simulink model "elsayed"  (R2023a)
settings: Solver=ode45  StartTime=0.0  StopTime=360  MaxStep=7.2  RelTol=1e-3
settings Model: Creator=Dell  LastModifiedBy=ENG-ELSAYED
settings SolverCC: MaxConsecutiveMinStep=10  AlgebraicLoopSolver=TrustRegion
settings DataIOCC: ReturnWorkspaceOutputs=off
settings DebuggingCC: UnconnectedInputMsg=warning  UnconnectedOutputMsg=warning  UnconnectedLineMsg=warning  ArithmeticOperatorsInVariantConditions=warning
settings ModelReferenceCC: EnableRefExpFcnMdlSchedulingChecks=on
settings SFSimCC: SimUseLocalCustomCode=off  CustomCodeUndefinedFunction=UseInterfaceOnly
settings RTWCC: RTWUseLocalCustomCode=off  DLArmComputeVersion=19.05

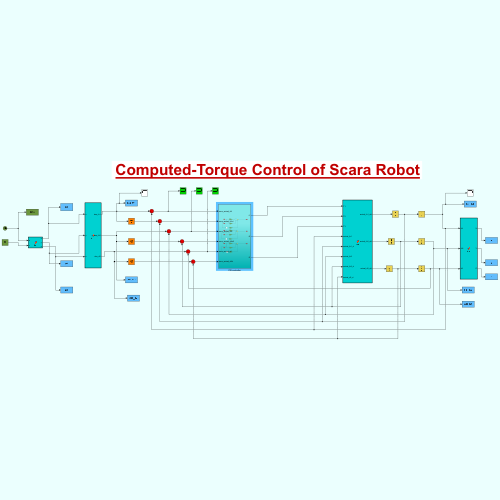
[thumbnail: Simulink's stored preview of the top-level diagram]
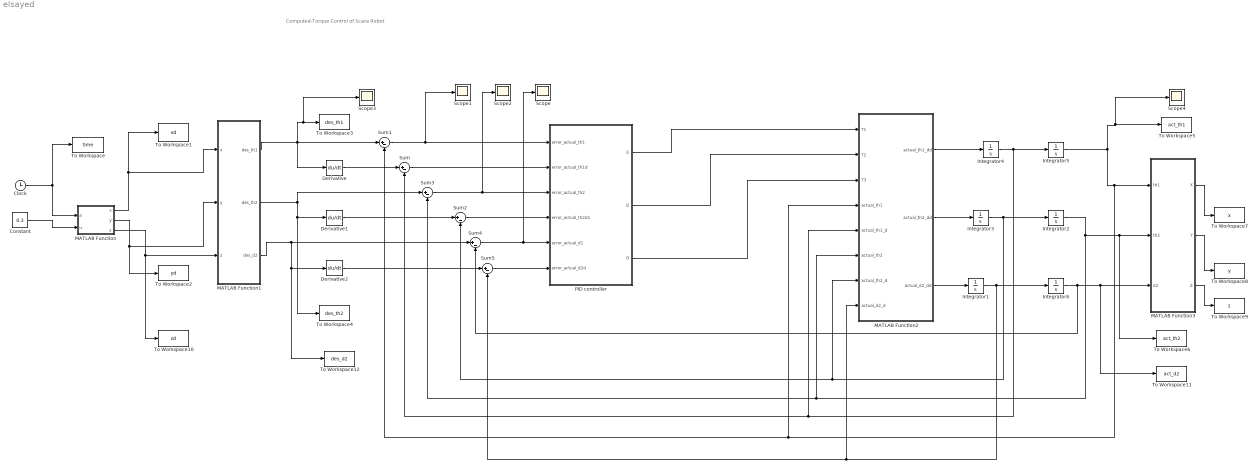
== system elsayed ==
  note: Computed-Torque Control of Scara Robot
  Clock : Clock
  Constant : Constant  Value=0.3
  Derivative : Derivative
  Derivative1 : Derivative
  Derivative2 : Derivative
  Integrator{1..6} (6 alike) : Integrator
  MATLAB Function : MATLAB Function  TreatAsAtomicUnit=on
  MATLAB Function1 : MATLAB Function  TreatAsAtomicUnit=on
  MATLAB Function2 : MATLAB Function  TreatAsAtomicUnit=on
  MATLAB Function3 : MATLAB Function  TreatAsAtomicUnit=on
  PID controller : Subsystem
  Scope{,1..4} (5 alike) : Scope
  Sum{,1..5} (6 alike) : Sum  Inputs=|+-
  To Workspace : ToWorkspace  VariableName=time  SampleTime=-1
  To Workspace1 : ToWorkspace  VariableName=xd  SampleTime=-1
  To Workspace10 : ToWorkspace  VariableName=zd  SampleTime=-1
      settings: Save2DSignal=2-D array (concatenate along first dimension)
  To Workspace11 : ToWorkspace  VariableName=act_d2  SampleTime=-1
  To Workspace12 : ToWorkspace  VariableName=des_d2  SampleTime=-1
  To Workspace2 : ToWorkspace  VariableName=yd  SampleTime=-1
      settings: Save2DSignal=2-D array (concatenate along first dimension)
  To Workspace3 : ToWorkspace  VariableName=des_th1  SampleTime=-1
  To Workspace4 : ToWorkspace  VariableName=des_th2  SampleTime=-1
  To Workspace5 : ToWorkspace  VariableName=act_th1  SampleTime=-1
  To Workspace6 : ToWorkspace  VariableName=act_th2  SampleTime=-1
  To Workspace7 : ToWorkspace  VariableName=x  SampleTime=-1
  To Workspace8 : ToWorkspace  VariableName=y  SampleTime=-1
  To Workspace9 : ToWorkspace  VariableName=z  SampleTime=-1
  wires:
  Clock/1 -> MATLAB Function/1(a), To Workspace/1
  MATLAB Function/1(x) -> MATLAB Function1/1(x), To Workspace1/1
  MATLAB Function/2(y) -> MATLAB Function1/2(y), To Workspace2/1
  MATLAB Function1/2(des_th2) -> To Workspace4/1, Derivative1/1, Sum3/1
  Derivative/1 -> Sum/1
  Derivative1/1 -> Sum2/1
  Sum/1 -> PID controller/2(error_actual_th1d)
  Sum3/1 -> Scope2/1, PID controller/3(error_actual_th2)
  Sum2/1 -> PID controller/4(error_actual_th2d1)
  PID controller/1(i1) -> MATLAB Function2/1(T1)
  PID controller/2(i2) -> MATLAB Function2/2(T2)
  MATLAB Function2/2(actual_th2_dd) -> Integrator3/1
  Integrator4/1 -> MATLAB Function2/5(actual_th1_d), Sum/2, Integrator5/1
  Integrator3/1 -> MATLAB Function2/7(actual_th2_d), Sum2/2, Integrator2/1
  Integrator5/1 -> MATLAB Function2/4(actual_th1), Sum1/2, MATLAB Function3/1(th1), Scope4/1, To Workspace5/1
  Integrator2/1 -> MATLAB Function2/6(actual_th2), Sum3/2, To Workspace6/1, MATLAB Function3/2(th2)
  MATLAB Function3/1(X) -> To Workspace7/1
  Sum1/1 -> Scope1/1, PID controller/1(error_actual_th1)
  Constant/1 -> MATLAB Function/2(u)
  MATLAB Function2/1(actual_th1_dd) -> Integrator4/1
  Sum4/1 -> Scope/1, PID controller/5(error_actual_d1)
  Derivative2/1 -> Sum5/1
  Sum5/1 -> PID controller/6(error_actual_d2d)
  PID controller/3(i3) -> MATLAB Function2/3(T3)
  MATLAB Function2/3(actual_d2_dd) -> Integrator1/1
  Integrator6/1 -> Sum4/2, To Workspace11/1, MATLAB Function3/3(d2)
  Integrator1/1 -> MATLAB Function2/8(actual_d2_d), Sum5/2, Integrator6/1
  MATLAB Function3/3(Z) -> To Workspace9/1
  MATLAB Function/3(z) -> MATLAB Function1/3(z), To Workspace10/1
  MATLAB Function1/1(des_th1) -> Derivative/1, Sum1/1, Scope3/1, To Workspace3/1
  MATLAB Function3/2(Y) -> To Workspace8/1
  MATLAB Function1/3(des_d2) -> To Workspace12/1, Derivative2/1, Sum4/1

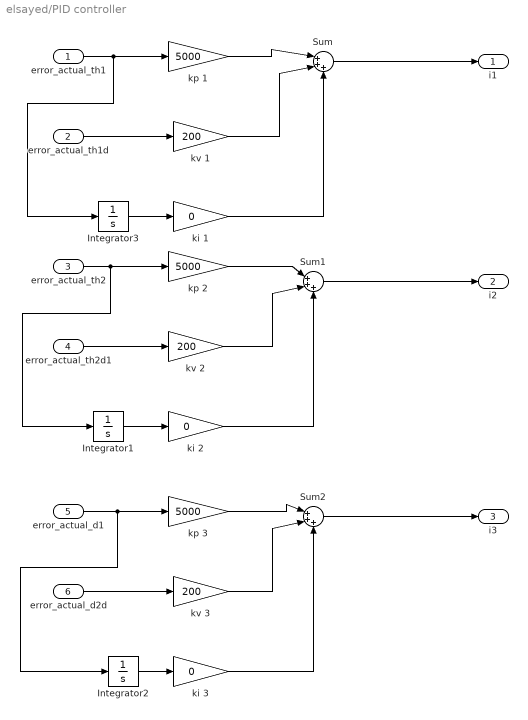
== system elsayed/PID controller ==
  error_actual_th1 : Inport
  error_actual_th1d : Inport  Port=2
  error_actual_th2 : Inport  Port=3
  error_actual_th2d1 : Inport  Port=4
  error_actual_d1 : Inport  Port=5
  error_actual_d2d : Inport  Port=6
  Integrator1 : Integrator
  Integrator2 : Integrator
  Integrator3 : Integrator
  Sum : Sum  Inputs=|+++
  Sum1 : Sum  Inputs=|+++
  Sum2 : Sum  Inputs=|+++
  ki 1 : Gain  Gain=0
  ki 2 : Gain  Gain=0
  ki 3 : Gain  Gain=0
  kp 1 : Gain  Gain=5000
  kp 2 : Gain  Gain=5000
  kp 3 : Gain  Gain=5000
  kv 1 : Gain  Gain=200
  kv 2 : Gain  Gain=200
  kv 3 : Gain  Gain=200
  i1 : Outport  VectorParamsAs1DForOutWhenUnconnected=off
  i2 : Outport  Port=2  VectorParamsAs1DForOutWhenUnconnected=off
  i3 : Outport  Port=3  VectorParamsAs1DForOutWhenUnconnected=off
  wires:
  Sum1/1 -> i2/1
  kp 2/1 -> Sum1/1
  kv 2/1 -> Sum1/2
  Sum2/1 -> i3/1
  kv 3/1 -> Sum2/2
  kp 3/1 -> Sum2/1
  Sum/1 -> i1/1
  kv 1/1 -> Sum/2
  kp 1/1 -> Sum/1
  error_actual_th1d/1 -> kv 1/1
  error_actual_th2d1/1 -> kv 2/1
  error_actual_d2d/1 -> kv 3/1
  Integrator1/1 -> ki 2/1
  error_actual_th2/1 -> Integrator1/1, kp 2/1
  ki 2/1 -> Sum1/3
  error_actual_d1/1 -> Integrator2/1, kp 3/1
  Integrator2/1 -> ki 3/1
  ki 3/1 -> Sum2/3
  Integrator3/1 -> ki 1/1
  error_actual_th1/1 -> Integrator3/1, kp 1/1
  ki 1/1 -> Sum/3

== matlab function elsayed/MATLAB Function1 ==
  data: x input; des_th1 output; y input; des_th2 output; des_d2 output; z input
function [des_th1, des_th2, des_d2] = fcn(x, y, z)
% Computes desired joint angles (des_th1, des_th2) and displacement (des_d2) 
% for a 2-link planar manipulator.

l1 = 2; % Length of first link
l2 = 2; % Length of second link
d1 = 2; % Offset along z-axis
d3 = 2; % Offset along z-axis
d4 = 2; % Offset along z-axis

% Calculate cos and sin of the second joint angle
c2 = (x^2 + y^2 - l1^2 - l2^2) / (2 * l1 * l2);
s2 = sqrt(1 - c2^2);

% Calculate the first joint angle
k1 = l1 + l2 * c2;
k2 = l2 * s2;
des_th1 = atan2(y, x) - atan2(k2, k1);

% Calculate the second joint angle
des_th2 = acos(c2);

% Calculate the linear displacement along z-axis
des_d2 = z - d1 + d3 + d4;
end

== matlab function elsayed/MATLAB Function ==
  data: a input; u input; x output; y output; z output
function [x,y,z] = fcn(a,u)
% FCN Computes the coordinates (x, y, z) based on input angle and distance.
% 
% Inputs:
%   a - Angle in degrees (scalar).
%   u - Distance or magnitude from the origin (scalar).

x = 1 + u*cosd(a); % Compute x-coordinate using cosine of angle a
y = 1 + u*sind(a); % Compute y-coordinate using sine of angle a
z = 8;             % Set z-coordinate to a constant value of 8
end

== matlab function elsayed/MATLAB Function2 ==
  data: actual_th1_dd output; actual_th2_dd output; T1 input; T2 input; T3 input; actual_th1 input; actual_th1_d input; actual_th2 input; actual_th2_d input; actual_d2_d input; actual_d2_dd output
function [actual_th1_dd, actual_th2_dd,actual_d2_dd] = fcn(T1,T2,T3, actual_th1,actual_th1_d,actual_th2,actual_th2_d,actual_d2_d)
m1=1; 
m2=1 ;
m3=1;
l1=2 ; 
l2=2  ;
I1= 0.001;
I2= 0.001 ;
I3=0.001;
g=9.81;
%Lc1=.5*L1;
%Lc2=.5*L2; 
th1 = actual_th1;
th2 = actual_th2;
th1d = actual_th1_d;
th2d = actual_th2_d;
%d2=actual_d2;
d2d=actual_d2_d;
M = [l1^2*m1/4+(m2*(4*l1^2+4*cos(th2)*l1*l2+l2^2))/4+0.5*(I1+I2+I3)  (l2*m2*(l2+2*l1*cos(th2)))/4+0.5*(I2) 0;
    (l2*m2*(l2+2*l1*cos(th2)))/4+ 0.5*(I2)                   (l2^2*m2)/4+0.5*(I2) 0;
    0                                                         0                    m1+m2+m3];

C= [-0.5*m2*l1*l2*sin(th2)*th2d   -0.5*m2*l1*l2*sin(th2)*(th2d) 0;
   0.5*m2*l1*l2*sin(th2)*th1d  -0.5*m2*l1*l2*sin(th2)*th1d 0;
   0                               0                       0];
V=C*[th1d;th2d;d2d];
G=[0.5*m1*g*l1*cos(th1)+(m2*g*(l1*cos(th1)+0.5*l2*cos(th1+th2)));
   0.5*m2*g*l2*cos(th1+th2);
   -g*(m1+m2+m3)];
T=[T1;T2;T3];
actual_th_dd= inv(M)*(T-V-G);
v=actual_th_dd(1);
w=actual_th_dd(2);
c=actual_th_dd(3);
actual_th1_dd =v;
actual_th2_dd= w;
actual_d2_dd=c;
end

== matlab function elsayed/MATLAB Function3 ==
  data: th1 input; X output; th2 input; Y output; d2 input; Z output
function [X,Y,Z]=fcn(th1,th2,d2)
l1=2;
l2=2;
d1=2;
d3=2;
d4=2;
X=l1*cos(th1)+l2*cos(th1+th2);
Y=l1*sin(th1)+l2*sin(th1+th2);
Z=d1+d2-d3-d4;
end
